simulink model "zad4"  (R2023b)
settings: Solver=VariableStepAuto  StartTime=0.0  StopTime=10  RelTol=1e-3
undefined symbols (not defined in the file or in its folder): start_x, start_y, tau, v
settings Model: Creator=student  LastModifiedBy=student

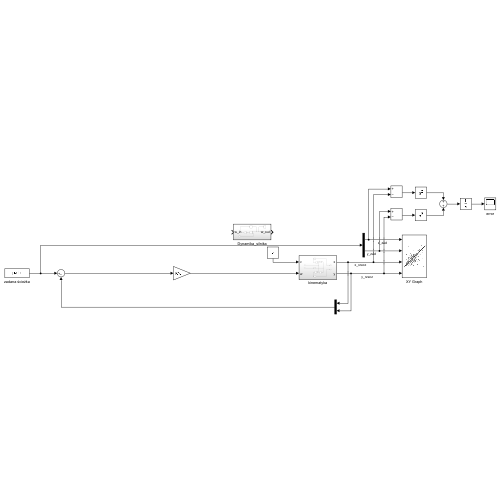
[thumbnail: Simulink's stored preview of the top-level diagram]
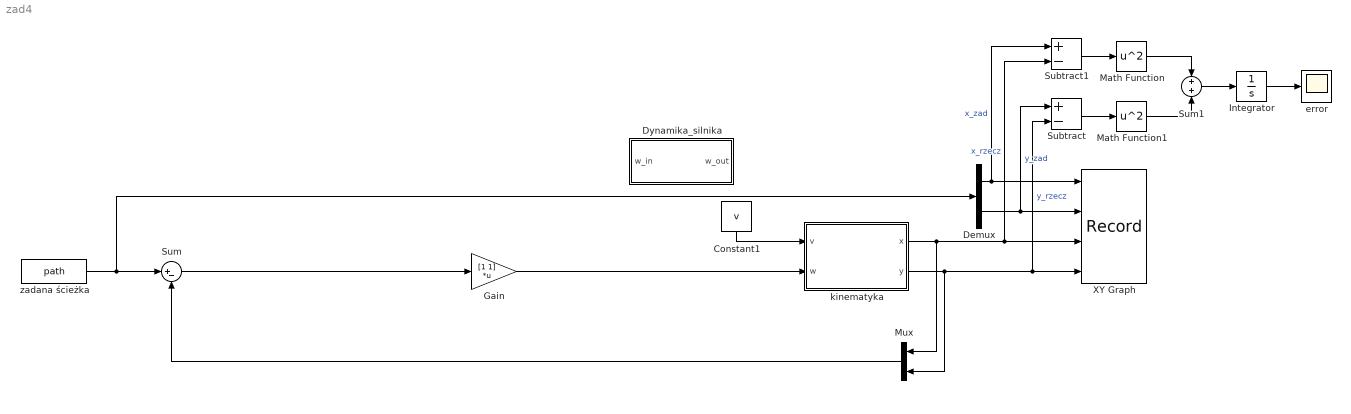
== system zad4 ==
  Constant1 : Constant  Value=v
  Demux : Demux  Outputs=2
  Dynamika_silnika : Subsystem
  Gain : Gain  Gain=[1 1]  Multiplication=Matrix(K*u)
  Integrator : Integrator
  Math Function : Math  Operator=square
  Math Function1 : Math  Operator=square
  Mux : Mux  Inputs=2
  Subtract : Sum  Inputs=+-
  Subtract1 : Sum  Inputs=+-
  Sum : Sum  Inputs=|+-
  Sum1 : Sum
  XY Graph : Record  FileSettingsInternal="{\"entries\":[{\"content\":{\"excelSettings\":{\"content\":{},\"type\":\"Streamout.ExcelSettings\"}},\"type\":\"Streamout.FileSettingStorage\",\"uuid\":\"\"}],\"packageUris\":[\"http:\\/\\/schema.mathworks.com\\/mf0\\/streamout_blocks\\/R2020a\"],\"version\":\"1.0\"}"  Layout=[1 1]  SignalsInternal="{\"entries\":[{\"content\":{\"signals\":[{\"content\":{\"blockPath\":[],\"dimensions\":[1],\"domain\":\"\",\"lineColor\":\"#77ac30\",\"plots\":[1],\"port\":1,\"sid\":[\"\"],\"signalID\":17848,\"signalName\":\"x_zad\"},\"type\":\"RecordBlkView.Signal\",\"uuid\":\"\"},{\"content\":{\"blockPath\":[],\"dimensions\":[1],\"domain\":\"\",\"lineColor\":\"#4dbeee\",\"plots\":[1],\"port\":2,\"sid\":[\"\"],\"signalID\":17852,\"signalName\":\"y_zad\"},\"type\":\"RecordBlkView.Signal\",\"uuid\":\"\"},{\"content\":{\"blockPath\":[],\"dimensions\":[1],\"domain\":\"\",\"lineColor\":\"#a2142f\",\"plots\":[1],\"port\":3,\"sid\":[\"\"],\"signalID\":17856,\"signalName\":\"x_rzecz\"},\"type\":\"RecordBlkView.Signal\",\"uuid\":\"\"},{\"content\":{\"blockPath\":[],\"dimensions\":[1],\"domain\":\"\",\"lineColor\":\"#139fff\",\"plots\":[1],\"port\":4,\"sid\":[\"\"],\"signalID\":17860,\"signalName\":\"y_rzecz\"},\"type\":\"RecordBlkView.Signal\",\"uuid\":\"\"}]},\"type\":\"RecordBlkView.InputSignals\",\"uuid\":\"\"}],\"packageUris\":[\"http:\\/\\/schema.mathworks.com\\/mf0\\/streamout_blocks\\/R2020a\"],\"version\":\"1.0\"}"  VisualizationBindings="{\"xyplotplugin\":{\"info\":[{\"series\":[{\"bindingParametersList\":[{\"parameter\":\"X-Axis\",\"signalID\":17848,\"signalName\":\"x_zad\"},{\"parameter\":\"Y-Axis\",\"signalID\":17852,\"signalName\":\"y_zad\"}],\"seriesID\":65483},{\"bindingParametersList\":[{\"parameter\":\"X-Axis\",\"signalID\":17860,\"signalName\":\"y_rzecz\"},{\"parameter\":\"Y-Axis\",\"signalID\":17856,\"signalName\":\"x_rzecz\"}],\"seriesID\":9649}],\"subplotID\":1}]}}"  CompatibilityTag=XY  st=-1
  error : Scope
  kinematyka : Subsystem
  "zadana ścieżka " : FromWorkspace  VariableName=path  OutDataTypeStr=double
  wires:
  kinematyka/1(x) -> Mux/1, Subtract1/2, XY Graph/3  "x_rzecz"
  kinematyka/2(y) -> Mux/2, Subtract/2, XY Graph/4  "y_rzecz"
  Demux/1 -> Subtract1/1, XY Graph/1  "x_zad"
  Demux/2 -> Subtract/1, XY Graph/2  "y_zad"
  Sum/1 -> Gain/1
  Subtract1/1 -> Math Function/1
  Subtract/1 -> Math Function1/1
  Math Function1/1 -> Sum1/2
  Math Function/1 -> Sum1/1
  Sum1/1 -> Integrator/1
  Integrator/1 -> error/1
  "zadana ścieżka "/1 -> Demux/1, Sum/1
  Mux/1 -> Sum/2
  Gain/1 -> kinematyka/2(w)
  Constant1/1 -> kinematyka/1(v)

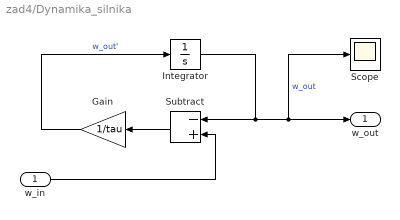
== system zad4/Dynamika_silnika ==
  w_in : Inport
  Gain : Gain  Gain=1/tau
  Integrator : Integrator
  Scope : Scope
  Subtract : Sum  Inputs=-+
  w_out : Outport
  wires:
  Gain/1 -> Integrator/1  "w_out'"
  Integrator/1 -> Scope/1, w_out/1, Subtract/1  "w_out"
  w_in/1 -> Subtract/2
  Subtract/1 -> Gain/1

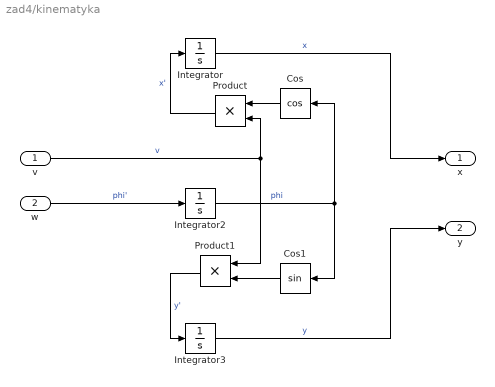
== system zad4/kinematyka ==
  v : Inport
  w : Inport  Port=2
  Cos : Trigonometry  Operator=cos
  Cos1 : Trigonometry
  Integrator : Integrator  InitialCondition=start_x
  Integrator2 : Integrator
  Integrator3 : Integrator  InitialCondition=start_y
  Product : Product
  Product1 : Product
  x : Outport
  y : Outport  Port=2
  wires:
  Integrator/1 -> x/1  "x"
  Product/1 -> Integrator/1  "x'"
  v/1 -> Product/2, Product1/1  "v"
  Integrator2/1 -> Cos1/1, Cos/1  "phi"
  w/1 -> Integrator2/1  "phi'"
  Cos/1 -> Product/1
  Product1/1 -> Integrator3/1  "y'"
  Integrator3/1 -> y/1  "y"
  Cos1/1 -> Product1/2
